simulink model "pv_array"  (Simulink 6.5)
settings: Solver=VariableStepDiscrete  StartTime=0.0  StopTime=1.0  MaxStep=0.005  RelTol=1e-3
libraries: simulink x9
settings Model: Creator=Mama  LastModifiedBy=Mama
settings DebuggingCC: AlgebraicLoopMsg=none  SolverPrmCheckMsg=none  UnconnectedOutputMsg=none

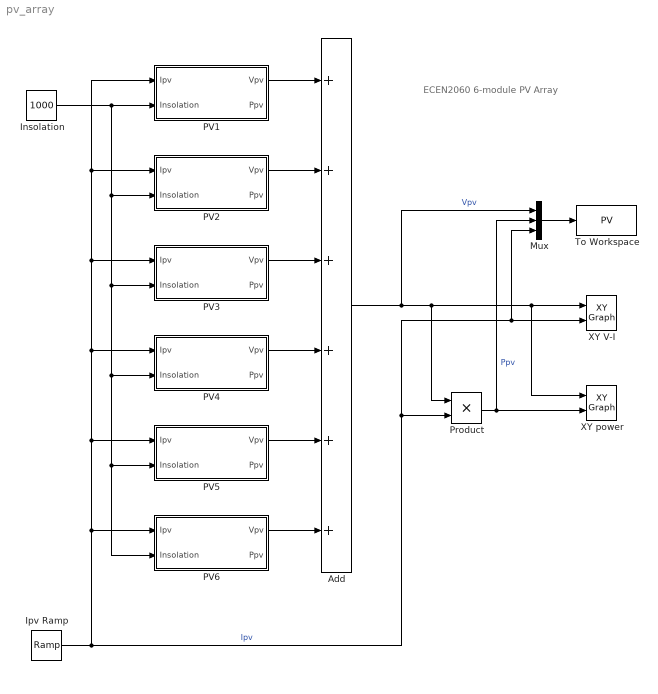
== system pv_array ==
  note: ECEN2060
      | 6-module PV Array
  Add : Sum  Inputs=++++++  OutScaling=2^-10
  Insolation : Constant  Value=1000  OutDataType=sfix(16)  ConRadixGroup=Use specified scaling  OutScaling=2^0  SampleTime=inf  FramePeriod=inf
  Ipv Ramp : simulink/Sources/Ramp  SystemSampleTime=-1  slope=6  start=0  X0=0
  Mux : Mux  Inputs=3
  PV1 : Subsystem  mask{Isc=5.45, Voc=22.2, Ir=4.95, Vr=17.2, Diode=on}
      mask prompts: Isc "Short-circuit current"; Voc "Open-circuit voltage"; Ir "Current at Pmax"; Vr "Voltage at Pmax"; Diode "By-pass diode?"
      mask help: PV module model based on module data-sheet parameters. This model has Ipv input, which is suitable for series connections. Limitations: no temperature dependance, static model
      mask init:
      | % calculation of PV module parameters
      | % limitation: constant temperature
      | Ns = round(Voc/0.61); % default number of cells in series
      | Vt = 26e-3; % thermal voltage
      | G = Isc/1000; % irradiation to short-circuit current gain
      | Vmpc = Vr/Ns; % cell voltage at rated Pmax
      | Vocc = Voc/Ns; % cell open-circuit voltage
      | Rmpp = Vmpc/Ir; % cell load resistance at Pmax
      | %
      | Rp = 100*Vocc/Isc; % initial value for Rp
      | Vdm = Vocc; % initial value for Vdm
      | %
      | % iterative solution for model parameters: Io, Rs, Rp
      | for i=1:10
      | %
      |  Idm = Isc - Ir - Vdm/Rp; % pn-junction (diode) current at MPP
      |  Io = (Isc-Vocc/Rp)/(exp(Vocc/Vt)-1); % pn-junction reverse saturation current
      |  Vdm = Vt*log(Idm/Io+1); % pn-junction (diode) voltage at MPP
      |  Rs = (Vdm-Vmpc)/Ir; % cell series resistance
      |  Rd = (Rmpp - Rs)*Rp/(Rp-Rmpp+Rs); % diode incremental resistance at MPP
      |  Idm = Vt/Rd; % diode current at MPP based on incremental resistance
      |  Rp = Vdm/(Isc-Ir-Idm); % cell parallel resistance
      | %
      | end
      | %
      mask Display:
      | plot([0.3 0.4],[0.4 0.8]);
      | plot([0.4 0.5],[0.4 0.8]);
      | plot([0.5 0.6],[0.4 0.8]);
      | plot([0.6 0.7],[0.4 0.8]);
      | plot([0.3 0.6],[0.4 0.4]);
      | plot([0.325 0.625],[0.5 0.5]);
      | plot([0.35 0.65],[0.6 0.6]);
      | plot([0.375 0.675],[0.7 0.7]);
      | plot([0.4 0.7],[0.8 0.8]);
      | text(0.5,0.9,'PV module (I)','horizontalAlignment', 'center');
  PV2 : Subsystem  mask{Isc=5.45, Voc=22.2, Ir=4.95, Vr=17.2, Diode=on}
      mask prompts: Isc "Short-circuit current"; Voc "Open-circuit voltage"; Ir "Current at Pmax"; Vr "Voltage at Pmax"; Diode "By-pass diode?"
      mask help: PV module model based on module data-sheet parameters. This model has Ipv input, which is suitable for series connections. Limitations: no temperature dependance, static model
      mask init: same as pv_array/PV1
      mask Display:
      | plot([0.3 0.4],[0.4 0.8]);
      | plot([0.4 0.5],[0.4 0.8]);
      | plot([0.5 0.6],[0.4 0.8]);
      | plot([0.6 0.7],[0.4 0.8]);
      | plot([0.3 0.6],[0.4 0.4]);
      | plot([0.325 0.625],[0.5 0.5]);
      | plot([0.35 0.65],[0.6 0.6]);
      | plot([0.375 0.675],[0.7 0.7]);
      | plot([0.4 0.7],[0.8 0.8]);
      | text(0.5,0.9,'PV module (I)','horizontalAlignment', 'center');
  PV3 : Subsystem  mask{Isc=5.45, Voc=22.2, Ir=4.95, Vr=17.2, Diode=on}
      mask prompts: Isc "Short-circuit current"; Voc "Open-circuit voltage"; Ir "Current at Pmax"; Vr "Voltage at Pmax"; Diode "By-pass diode?"
      mask help: PV module model based on module data-sheet parameters. This model has Ipv input, which is suitable for series connections. Limitations: no temperature dependance, static model
      mask init: same as pv_array/PV1
      mask Display:
      | plot([0.3 0.4],[0.4 0.8]);
      | plot([0.4 0.5],[0.4 0.8]);
      | plot([0.5 0.6],[0.4 0.8]);
      | plot([0.6 0.7],[0.4 0.8]);
      | plot([0.3 0.6],[0.4 0.4]);
      | plot([0.325 0.625],[0.5 0.5]);
      | plot([0.35 0.65],[0.6 0.6]);
      | plot([0.375 0.675],[0.7 0.7]);
      | plot([0.4 0.7],[0.8 0.8]);
      | text(0.5,0.9,'PV module (I)','horizontalAlignment', 'center');
  PV4 : Subsystem  mask{Isc=5.45, Voc=22.2, Ir=4.95, Vr=17.2, Diode=on}
      mask prompts: Isc "Short-circuit current"; Voc "Open-circuit voltage"; Ir "Current at Pmax"; Vr "Voltage at Pmax"; Diode "By-pass diode?"
      mask help: PV module model based on module data-sheet parameters. This model has Ipv input, which is suitable for series connections. Limitations: no temperature dependance, static model
      mask init: same as pv_array/PV1
      mask Display:
      | plot([0.3 0.4],[0.4 0.8]);
      | plot([0.4 0.5],[0.4 0.8]);
      | plot([0.5 0.6],[0.4 0.8]);
      | plot([0.6 0.7],[0.4 0.8]);
      | plot([0.3 0.6],[0.4 0.4]);
      | plot([0.325 0.625],[0.5 0.5]);
      | plot([0.35 0.65],[0.6 0.6]);
      | plot([0.375 0.675],[0.7 0.7]);
      | plot([0.4 0.7],[0.8 0.8]);
      | text(0.5,0.9,'PV module (I)','horizontalAlignment', 'center');
  PV5 : Subsystem  mask{Isc=5.45, Voc=22.2, Ir=4.95, Vr=17.2, Diode=on}
      mask prompts: Isc "Short-circuit current"; Voc "Open-circuit voltage"; Ir "Current at Pmax"; Vr "Voltage at Pmax"; Diode "By-pass diode?"
      mask help: PV module model based on module data-sheet parameters. This model has Ipv input, which is suitable for series connections. Limitations: no temperature dependance, static model
      mask init: same as pv_array/PV1
      mask Display:
      | plot([0.3 0.4],[0.4 0.8]);
      | plot([0.4 0.5],[0.4 0.8]);
      | plot([0.5 0.6],[0.4 0.8]);
      | plot([0.6 0.7],[0.4 0.8]);
      | plot([0.3 0.6],[0.4 0.4]);
      | plot([0.325 0.625],[0.5 0.5]);
      | plot([0.35 0.65],[0.6 0.6]);
      | plot([0.375 0.675],[0.7 0.7]);
      | plot([0.4 0.7],[0.8 0.8]);
      | text(0.5,0.9,'PV module (I)','horizontalAlignment', 'center');
  PV6 : Subsystem  mask{Isc=5.45, Voc=22.2, Ir=4.95, Vr=17.2, Diode=on}
      mask prompts: Isc "Short-circuit current"; Voc "Open-circuit voltage"; Ir "Current at Pmax"; Vr "Voltage at Pmax"; Diode "By-pass diode?"
      mask help: PV module model based on module data-sheet parameters. This model has Ipv input, which is suitable for series connections. Limitations: no temperature dependance, static model
      mask init: same as pv_array/PV1
      mask Display:
      | plot([0.3 0.4],[0.4 0.8]);
      | plot([0.4 0.5],[0.4 0.8]);
      | plot([0.5 0.6],[0.4 0.8]);
      | plot([0.6 0.7],[0.4 0.8]);
      | plot([0.3 0.6],[0.4 0.4]);
      | plot([0.325 0.625],[0.5 0.5]);
      | plot([0.35 0.65],[0.6 0.6]);
      | plot([0.375 0.675],[0.7 0.7]);
      | plot([0.4 0.7],[0.8 0.8]);
      | text(0.5,0.9,'PV module (I)','horizontalAlignment', 'center');
  Product : Product  RndMeth=Zero
  To Workspace : ToWorkspace  VariableName=PV  SampleTime=-1  SaveFormat=Structure With Time
  XY V-I : simulink/Sinks/XY Graph  SystemSampleTime=-1  xmin=0  xmax=150  ymin=0  ymax=6  st=-1
  XY power : simulink/Sinks/XY Graph  SystemSampleTime=-1  xmin=0  xmax=150  ymin=0  ymax=600  st=-1
  wires:
  Ipv Ramp/1 -> PV1/1(Ipv), PV2/1(Ipv), PV3/1(Ipv), PV4/1(Ipv), PV5/1(Ipv), PV6/1(Ipv), Product/2, XY V-I/2, Mux/3  "Ipv"
  Mux/1 -> To Workspace/1
  PV1/1(Vpv) -> Add/1
  PV2/1(Vpv) -> Add/2
  PV3/1(Vpv) -> Add/3
  PV4/1(Vpv) -> Add/4
  PV5/1(Vpv) -> Add/5
  PV6/1(Vpv) -> Add/6
  Add/1 -> XY V-I/1, XY power/1, Product/1, Mux/1  "Vpv"
  Insolation/1 -> PV5/2(Insolation), PV6/2(Insolation), PV4/2(Insolation), PV3/2(Insolation), PV2/2(Insolation), PV1/2(Insolation)
  Product/1 -> XY power/2, Mux/2  "Ppv"

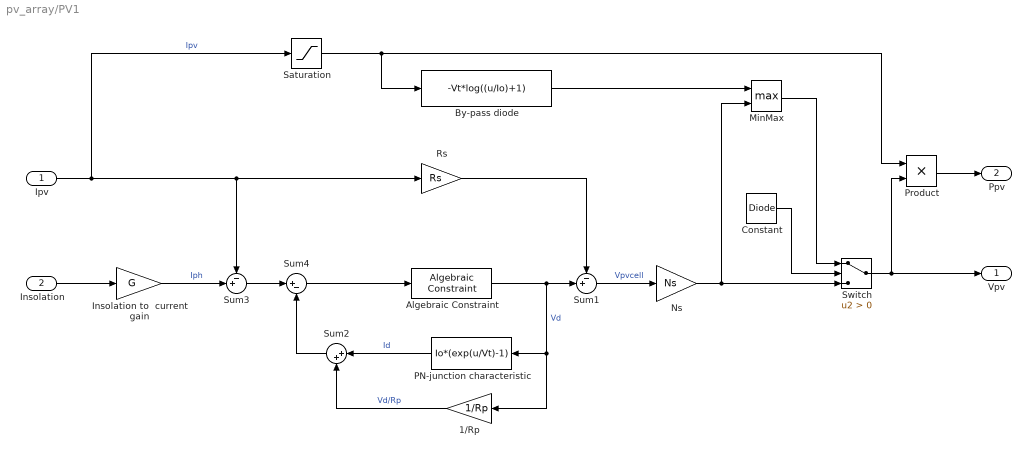
== system pv_array/PV1 ==
  Ipv : Inport
  Insolation : Inport  Port=2
  1/Rp : Gain  Orientation=left  Gain=1/Rp
  Algebraic Constraint : simulink/Math Operations/Algebraic Constraint  SystemSampleTime=-1  z0=0
  By-pass diode : Fcn  Expr=-Vt*log((u/Io)+1)
  Constant : Constant  Value=Diode  OutDataType=sfix(16)  ConRadixGroup=Use specified scaling  OutScaling=2^0  SampleTime=inf  FramePeriod=inf
  Insolation to  current gain : Gain  Gain=G
  MinMax : MinMax  Function=max  Inputs=2
  Ns : Gain  Gain=Ns
  PN-junction characteristic : Fcn  Orientation=left  Expr=Io*(exp(u/Vt)-1)
  Product : Product  RndMeth=Zero
  Rs : Gain  Gain=Rs
  Saturation : Saturate  UpperLimit=inf  LowerLimit=0
  Sum1 : Sum  Inputs=-+|
  Sum2 : Sum  Orientation=left  Inputs=|++
  Sum3 : Sum  Inputs=-+|
  Sum4 : Sum  Inputs=|+-
  Switch : Switch  Criteria=u2 > Threshold
  Vpv : Outport
  Ppv : Outport  Port=2
  wires:
  Insolation/1 -> Insolation to  current gain/1
  Insolation to  current gain/1 -> Sum3/2  "Iph"
  Ipv/1 -> Saturation/1, Sum3/1, Rs/1  "Ipv"
  Product/1 -> Ppv/1
  Sum4/1 -> Algebraic Constraint/1
  Algebraic Constraint/1 -> Sum1/2, 1/Rp/1, PN-junction characteristic/1  "Vd"
  Sum1/1 -> Ns/1  "Vpvcell"
  Rs/1 -> Sum1/1
  By-pass diode/1 -> MinMax/1
  Ns/1 -> MinMax/2, Switch/3
  MinMax/1 -> Switch/1
  Constant/1 -> Switch/2
  Switch/1 -> Vpv/1, Product/2
  Saturation/1 -> Product/1, By-pass diode/1
  Sum3/1 -> Sum4/1
  Sum2/1 -> Sum4/2
  PN-junction characteristic/1 -> Sum2/1  "Id"
  1/Rp/1 -> Sum2/2  "Vd/Rp"

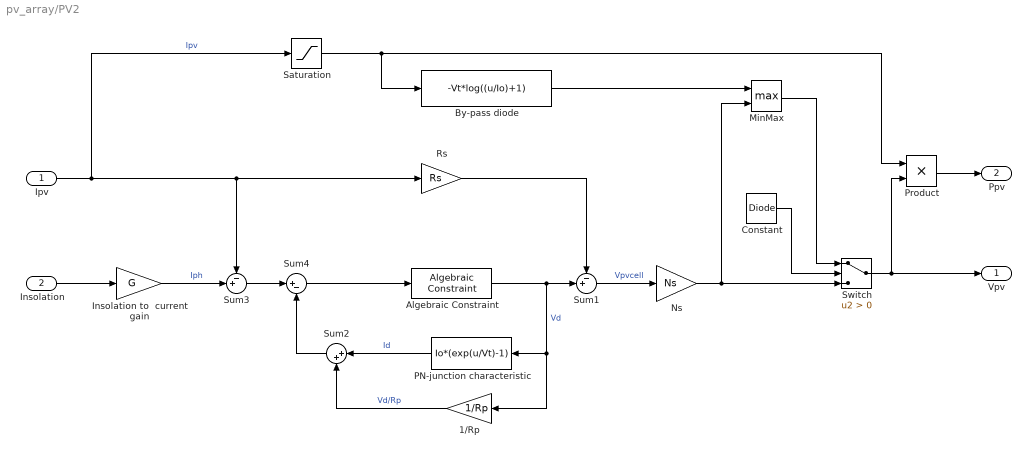
== system pv_array/PV2 ==
  Ipv : Inport
  Insolation : Inport  Port=2
  1/Rp : Gain  Orientation=left  Gain=1/Rp
  Algebraic Constraint : simulink/Math Operations/Algebraic Constraint  SystemSampleTime=-1  z0=0
  By-pass diode : Fcn  Expr=-Vt*log((u/Io)+1)
  Constant : Constant  Value=Diode  OutDataType=sfix(16)  ConRadixGroup=Use specified scaling  OutScaling=2^0  SampleTime=inf  FramePeriod=inf
  Insolation to  current gain : Gain  Gain=G
  MinMax : MinMax  Function=max  Inputs=2
  Ns : Gain  Gain=Ns
  PN-junction characteristic : Fcn  Orientation=left  Expr=Io*(exp(u/Vt)-1)
  Product : Product  RndMeth=Zero
  Rs : Gain  Gain=Rs
  Saturation : Saturate  UpperLimit=inf  LowerLimit=0
  Sum1 : Sum  Inputs=-+|
  Sum2 : Sum  Orientation=left  Inputs=|++
  Sum3 : Sum  Inputs=-+|
  Sum4 : Sum  Inputs=|+-
  Switch : Switch  Criteria=u2 > Threshold
  Vpv : Outport
  Ppv : Outport  Port=2
  wires:
  Insolation/1 -> Insolation to  current gain/1
  Insolation to  current gain/1 -> Sum3/2  "Iph"
  Ipv/1 -> Saturation/1, Sum3/1, Rs/1  "Ipv"
  Product/1 -> Ppv/1
  Sum4/1 -> Algebraic Constraint/1
  Algebraic Constraint/1 -> Sum1/2, 1/Rp/1, PN-junction characteristic/1  "Vd"
  Sum1/1 -> Ns/1  "Vpvcell"
  Rs/1 -> Sum1/1
  By-pass diode/1 -> MinMax/1
  Ns/1 -> MinMax/2, Switch/3
  MinMax/1 -> Switch/1
  Constant/1 -> Switch/2
  Switch/1 -> Vpv/1, Product/2
  Saturation/1 -> Product/1, By-pass diode/1
  Sum3/1 -> Sum4/1
  Sum2/1 -> Sum4/2
  PN-junction characteristic/1 -> Sum2/1  "Id"
  1/Rp/1 -> Sum2/2  "Vd/Rp"

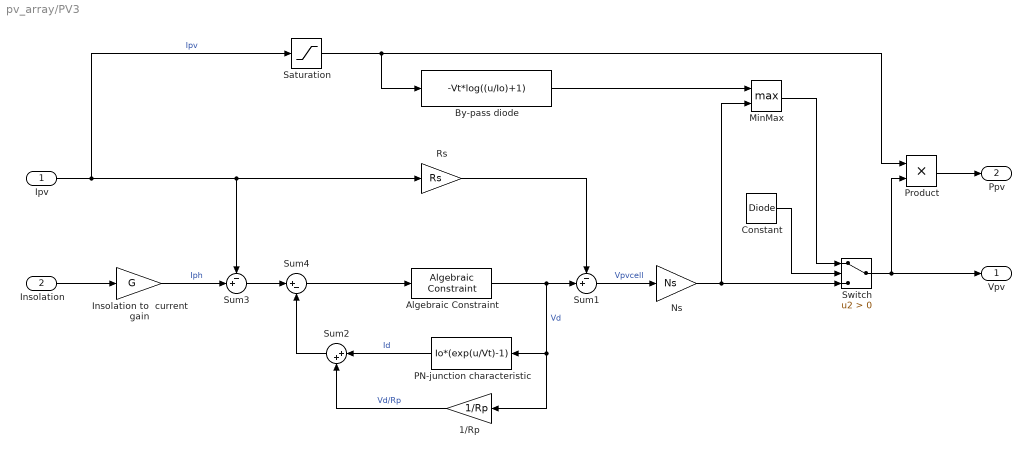
== system pv_array/PV3 ==
  Ipv : Inport
  Insolation : Inport  Port=2
  1/Rp : Gain  Orientation=left  Gain=1/Rp
  Algebraic Constraint : simulink/Math Operations/Algebraic Constraint  SystemSampleTime=-1  z0=0
  By-pass diode : Fcn  Expr=-Vt*log((u/Io)+1)
  Constant : Constant  Value=Diode  OutDataType=sfix(16)  ConRadixGroup=Use specified scaling  OutScaling=2^0  SampleTime=inf  FramePeriod=inf
  Insolation to  current gain : Gain  Gain=G
  MinMax : MinMax  Function=max  Inputs=2
  Ns : Gain  Gain=Ns
  PN-junction characteristic : Fcn  Orientation=left  Expr=Io*(exp(u/Vt)-1)
  Product : Product  RndMeth=Zero
  Rs : Gain  Gain=Rs
  Saturation : Saturate  UpperLimit=inf  LowerLimit=0
  Sum1 : Sum  Inputs=-+|
  Sum2 : Sum  Orientation=left  Inputs=|++
  Sum3 : Sum  Inputs=-+|
  Sum4 : Sum  Inputs=|+-
  Switch : Switch  Criteria=u2 > Threshold
  Vpv : Outport
  Ppv : Outport  Port=2
  wires:
  Insolation/1 -> Insolation to  current gain/1
  Insolation to  current gain/1 -> Sum3/2  "Iph"
  Ipv/1 -> Saturation/1, Sum3/1, Rs/1  "Ipv"
  Product/1 -> Ppv/1
  Sum4/1 -> Algebraic Constraint/1
  Algebraic Constraint/1 -> Sum1/2, 1/Rp/1, PN-junction characteristic/1  "Vd"
  Sum1/1 -> Ns/1  "Vpvcell"
  Rs/1 -> Sum1/1
  By-pass diode/1 -> MinMax/1
  Ns/1 -> MinMax/2, Switch/3
  MinMax/1 -> Switch/1
  Constant/1 -> Switch/2
  Switch/1 -> Vpv/1, Product/2
  Saturation/1 -> Product/1, By-pass diode/1
  Sum3/1 -> Sum4/1
  Sum2/1 -> Sum4/2
  PN-junction characteristic/1 -> Sum2/1  "Id"
  1/Rp/1 -> Sum2/2  "Vd/Rp"

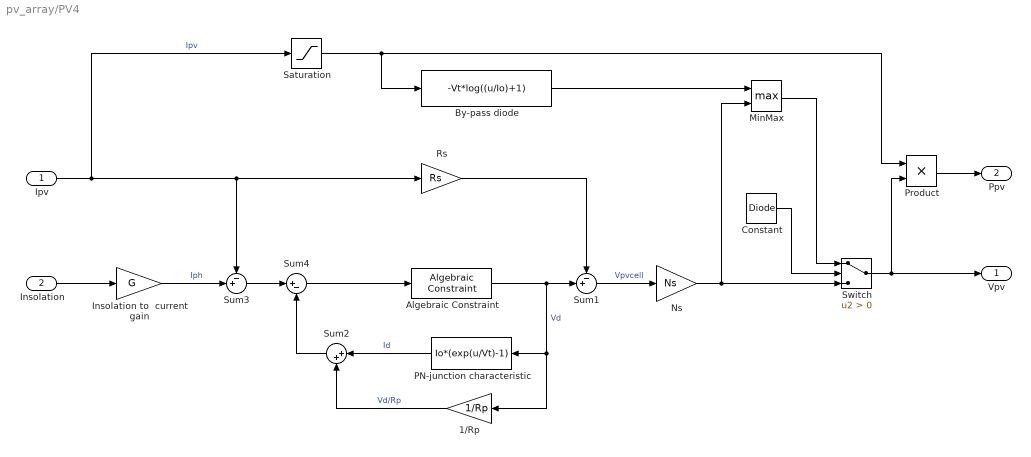
== system pv_array/PV4 ==
  Ipv : Inport
  Insolation : Inport  Port=2
  1/Rp : Gain  Orientation=left  Gain=1/Rp
  Algebraic Constraint : simulink/Math Operations/Algebraic Constraint  SystemSampleTime=-1  z0=0
  By-pass diode : Fcn  Expr=-Vt*log((u/Io)+1)
  Constant : Constant  Value=Diode  OutDataType=sfix(16)  ConRadixGroup=Use specified scaling  OutScaling=2^0  SampleTime=inf  FramePeriod=inf
  Insolation to  current gain : Gain  Gain=G
  MinMax : MinMax  Function=max  Inputs=2
  Ns : Gain  Gain=Ns
  PN-junction characteristic : Fcn  Orientation=left  Expr=Io*(exp(u/Vt)-1)
  Product : Product  RndMeth=Zero
  Rs : Gain  Gain=Rs
  Saturation : Saturate  UpperLimit=inf  LowerLimit=0
  Sum1 : Sum  Inputs=-+|
  Sum2 : Sum  Orientation=left  Inputs=|++
  Sum3 : Sum  Inputs=-+|
  Sum4 : Sum  Inputs=|+-
  Switch : Switch  Criteria=u2 > Threshold
  Vpv : Outport
  Ppv : Outport  Port=2
  wires:
  Insolation/1 -> Insolation to  current gain/1
  Insolation to  current gain/1 -> Sum3/2  "Iph"
  Ipv/1 -> Saturation/1, Sum3/1, Rs/1  "Ipv"
  Product/1 -> Ppv/1
  Sum4/1 -> Algebraic Constraint/1
  Algebraic Constraint/1 -> Sum1/2, 1/Rp/1, PN-junction characteristic/1  "Vd"
  Sum1/1 -> Ns/1  "Vpvcell"
  Rs/1 -> Sum1/1
  By-pass diode/1 -> MinMax/1
  Ns/1 -> MinMax/2, Switch/3
  MinMax/1 -> Switch/1
  Constant/1 -> Switch/2
  Switch/1 -> Vpv/1, Product/2
  Saturation/1 -> Product/1, By-pass diode/1
  Sum3/1 -> Sum4/1
  Sum2/1 -> Sum4/2
  PN-junction characteristic/1 -> Sum2/1  "Id"
  1/Rp/1 -> Sum2/2  "Vd/Rp"

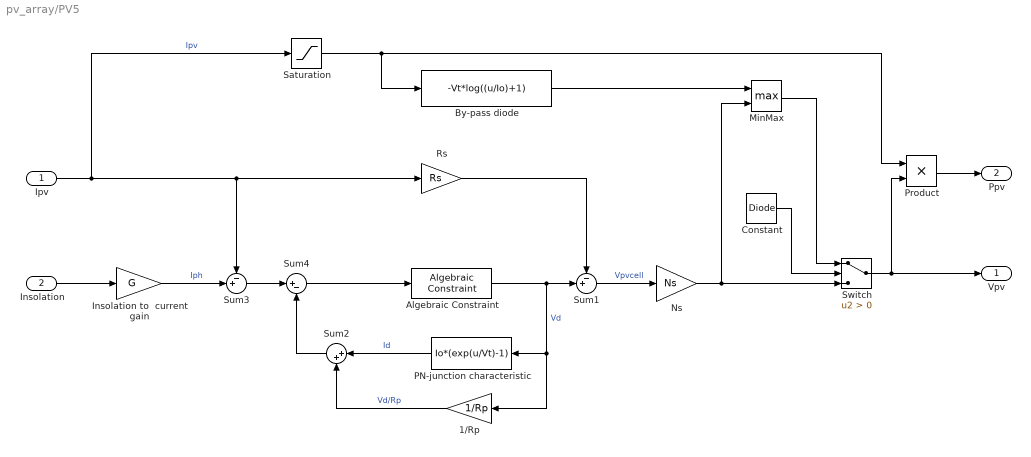
== system pv_array/PV5 ==
  Ipv : Inport
  Insolation : Inport  Port=2
  1/Rp : Gain  Orientation=left  Gain=1/Rp
  Algebraic Constraint : simulink/Math Operations/Algebraic Constraint  SystemSampleTime=-1  z0=0
  By-pass diode : Fcn  Expr=-Vt*log((u/Io)+1)
  Constant : Constant  Value=Diode  OutDataType=sfix(16)  ConRadixGroup=Use specified scaling  OutScaling=2^0  SampleTime=inf  FramePeriod=inf
  Insolation to  current gain : Gain  Gain=G
  MinMax : MinMax  Function=max  Inputs=2
  Ns : Gain  Gain=Ns
  PN-junction characteristic : Fcn  Orientation=left  Expr=Io*(exp(u/Vt)-1)
  Product : Product  RndMeth=Zero
  Rs : Gain  Gain=Rs
  Saturation : Saturate  UpperLimit=inf  LowerLimit=0
  Sum1 : Sum  Inputs=-+|
  Sum2 : Sum  Orientation=left  Inputs=|++
  Sum3 : Sum  Inputs=-+|
  Sum4 : Sum  Inputs=|+-
  Switch : Switch  Criteria=u2 > Threshold
  Vpv : Outport
  Ppv : Outport  Port=2
  wires:
  Insolation/1 -> Insolation to  current gain/1
  Insolation to  current gain/1 -> Sum3/2  "Iph"
  Ipv/1 -> Saturation/1, Sum3/1, Rs/1  "Ipv"
  Product/1 -> Ppv/1
  Sum4/1 -> Algebraic Constraint/1
  Algebraic Constraint/1 -> Sum1/2, 1/Rp/1, PN-junction characteristic/1  "Vd"
  Sum1/1 -> Ns/1  "Vpvcell"
  Rs/1 -> Sum1/1
  By-pass diode/1 -> MinMax/1
  Ns/1 -> MinMax/2, Switch/3
  MinMax/1 -> Switch/1
  Constant/1 -> Switch/2
  Switch/1 -> Vpv/1, Product/2
  Saturation/1 -> Product/1, By-pass diode/1
  Sum3/1 -> Sum4/1
  Sum2/1 -> Sum4/2
  PN-junction characteristic/1 -> Sum2/1  "Id"
  1/Rp/1 -> Sum2/2  "Vd/Rp"

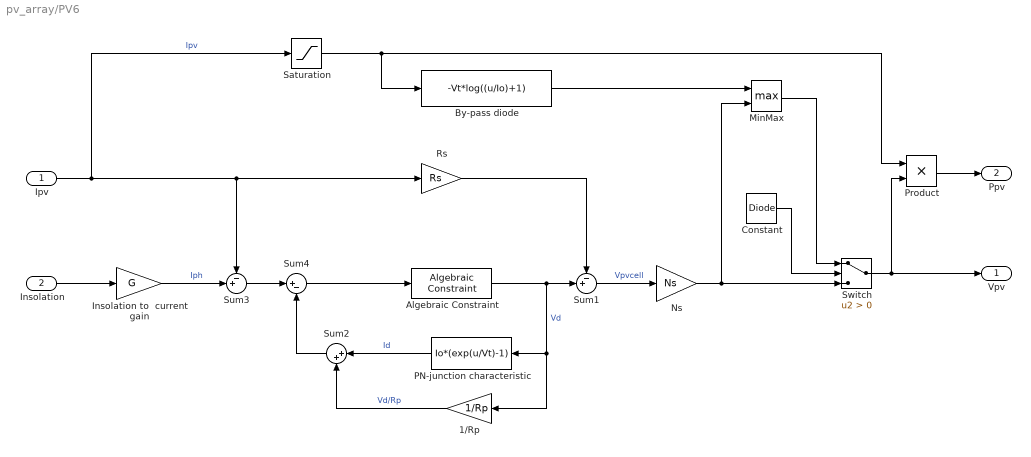
== system pv_array/PV6 ==
  Ipv : Inport
  Insolation : Inport  Port=2
  1/Rp : Gain  Orientation=left  Gain=1/Rp
  Algebraic Constraint : simulink/Math Operations/Algebraic Constraint  SystemSampleTime=-1  z0=0
  By-pass diode : Fcn  Expr=-Vt*log((u/Io)+1)
  Constant : Constant  Value=Diode  OutDataType=sfix(16)  ConRadixGroup=Use specified scaling  OutScaling=2^0  SampleTime=inf  FramePeriod=inf
  Insolation to  current gain : Gain  Gain=G
  MinMax : MinMax  Function=max  Inputs=2
  Ns : Gain  Gain=Ns
  PN-junction characteristic : Fcn  Orientation=left  Expr=Io*(exp(u/Vt)-1)
  Product : Product  RndMeth=Zero
  Rs : Gain  Gain=Rs
  Saturation : Saturate  UpperLimit=inf  LowerLimit=0
  Sum1 : Sum  Inputs=-+|
  Sum2 : Sum  Orientation=left  Inputs=|++
  Sum3 : Sum  Inputs=-+|
  Sum4 : Sum  Inputs=|+-
  Switch : Switch  Criteria=u2 > Threshold
  Vpv : Outport
  Ppv : Outport  Port=2
  wires:
  Insolation/1 -> Insolation to  current gain/1
  Insolation to  current gain/1 -> Sum3/2  "Iph"
  Ipv/1 -> Saturation/1, Sum3/1, Rs/1  "Ipv"
  Product/1 -> Ppv/1
  Sum4/1 -> Algebraic Constraint/1
  Algebraic Constraint/1 -> Sum1/2, 1/Rp/1, PN-junction characteristic/1  "Vd"
  Sum1/1 -> Ns/1  "Vpvcell"
  Rs/1 -> Sum1/1
  By-pass diode/1 -> MinMax/1
  Ns/1 -> MinMax/2, Switch/3
  MinMax/1 -> Switch/1
  Constant/1 -> Switch/2
  Switch/1 -> Vpv/1, Product/2
  Saturation/1 -> Product/1, By-pass diode/1
  Sum3/1 -> Sum4/1
  Sum2/1 -> Sum4/2
  PN-junction characteristic/1 -> Sum2/1  "Id"
  1/Rp/1 -> Sum2/2  "Vd/Rp"
